simulink model "nms3D_2021"  (R2021a)
settings: Solver=ode15s  StartTime=0.0  StopTime=2  MaxStep=1e-2  RelTol=1e-2
StartFcn:
  | tic
StopFcn:
  | toc
  | 
  | 
  | %if GimbalLockFlag
  |  % fprintf(2, 'Almost reached Gimbal Lock of IMU. Simulation stopped.\n')
  | %end
  | 
  | %fprintf('Elapsed time: %4.2f sec (%4.2f%% realtime)\n', a, tout(end)/a*100)
values from neighbouring files (symbols this model uses):
  Balance02 = pMod(24:29)    [AssignSimulinkParams.m]    (also in assign_parameters.m = param(26:29))
  Balance13 = pMod(30:35)    [AssignSimulinkParams.m]    (also in assign_parameters.m = param(30:33))
  BalanceTrunk = pMod(22:23)    [AssignSimulinkParams.m]    (also in assign_parameters.m = param(22:23))
  BalanceTrunkLat = param(24:25)    [assign_parameters.m]
  BalanceTrunkLatOld = pMod(43:46)    [AssignSimulinkParams.m]    (also in assign_parameters.m = param(43:46))
  BalanceTrunkOld = param(49:53)    [assign_parameters.m]
  BasisStim = pMod(1:11)    [AssignSimulinkParams.m]    (also in assign_parameters.m = param(1:11))
  CompliantLeg = pMod(12:14)    [AssignSimulinkParams.m]    (also in assign_parameters.m = param(12:14))
  CompliantLegLat = pMod(15)    [AssignSimulinkParams.m]    (also in assign_parameters.m = param(15))
  PreventKneeOverextension = pMod(16:21)    [AssignSimulinkParams.m]    (also in assign_parameters.m = param(16:21))
  SwingCompLatOld = param(47:48)    [assign_parameters.m]
  Target02 = pMod(36:38)    [AssignSimulinkParams.m]    (also in assign_parameters.m = param(34:36))
  Target02_va = pMod(49:54)    [AssignSimulinkParams.m]    (also in assign_parameters.m = param(60:65))
  Target13 = pMod(39:41)    [AssignSimulinkParams.m]    (also in assign_parameters.m = param(37:39))
  Target13_va = pMod(55:60)    [AssignSimulinkParams.m]    (also in assign_parameters.m = param(66:71))
  theta0_world = param(59)    [assign_parameters.m]
  WramameiSL_1000 = readmatrix('WSL_1000_Norm_Sigmoid_MSE_cont.csv')    [nms3D_prep.m]
  ZramameiSL_1000 = readmatrix('ZSL_1000_Norm_Sigmoid_MSE_cont.csv')    [nms3D_prep.m]
undefined symbols (not defined in the file or in its folder): ICs, mParams, X, Y, Z
libraries: nesl_utility x106, sm_lib x87, simulink x70, eeGeneralControl x28, robotmaniplib x14, dspinverses x10, robotcorelib x5, dspmathops x3, vrlib x1, pid_lib x1
(part 1 of 8)
settings Model: Creator=hgeyer  LastModifiedBy=rachidramadan
settings SolverCC: AlgebraicLoopSolver=TrustRegion  MinimalZcImpactIntegration=on
settings OptimizationCC: EfficientMapNaN2IntZero=off
settings DebuggingCC: ReadBeforeWriteMsg=DisableAll  WriteAfterWriteMsg=DisableAll  WriteAfterReadMsg=DisableAll  IgnoredZcDiagnostic=none  MultiTaskDSMMsg=none  SFMachineParentedDataDiag=warning  ArithmeticOperatorsInVariantConditions=warning
settings HardwareCC: TargetBitPerLong=64  TargetBitPerPointer=64  TargetBitPerSizeT=64  TargetBitPerPtrDiffT=64  TargetLongLongMode=on  TargetIntDivRoundTo=Zero  TargetEndianess=LittleEndian  TargetWordSize=64  TargetHWDeviceType=MATLAB Host  ProdEqTarget=off
settings ModelReferenceCC: UpdateModelReferenceTargets=IfOutOfDate
settings SFSimCC: SFSimEcho=off  SimUseLocalCustomCode=off  CustomCodeUndefinedFunction=UseInterfaceOnly
settings CodeAppCC: MaxIdLength=128
settings ConfigComp: CovScope=ReferencedModels
settings SimscapeCC: SimscapeNormalizeSystem=off
settings ExplorerConfigSet: InternalSimMechanicsExplorerSettings="<ExplorerConfiguration><canonicalview>planar_xy</canonicalview><AnimationSetting><BasePlaybackSpeed>1.0</BasePlaybackSpeed><PlaybackSpeedFactor>1.0</PlaybackSpeedFactor></AnimationSetting><TilePanel><TileInfo><Tiles Columns=\"1\" Count=\"1\" Rows=\"1\"><Column Weight=\"1\"/><Row Weight=\"1\"/><Tile Height=\"1\" Width=\"1\" X=\"0\" Y=\"0\"/></Tiles></TileInfo><SceneInfo><SceneViewer><BGColor><R>0.60000002384185791</R><G>0.60000002384185791</G><B>0.60000002384185791</B></BGColor><Camera><DoPerspective>off</DoPerspective><Position><X>0.597774143722594631</X><Y>0.919449529340500282</Y><Z>14.1815791267909113</Z></Position><Center><X>0.597774143722594631</X><Y>0.919449529340500282</Y><Z>3.38181724401920292e-07</Z></Center><Up><X>0</X><Y>1</Y><Z>0</Z></Up><ViewLimDist>1</ViewLimDist><YLim>1.30566284997374105</YLim><XLim>1.60885047805753101</XLim></Camera></SceneViewer></SceneInfo></TilePanel><MechEditorPanel><Cameras/><GfxPanelCameraMap/><VideoCreator><PlaybackSpeedRatio>1.0</PlaybackSpeedRatio><FrameRate>30</FrameRate><VideoFormat>Motion JPEG AVI</VideoFormat><FrameSize>auto</FrameSize></VideoCreator></MechEditorPanel></ExplorerConfiguration>"

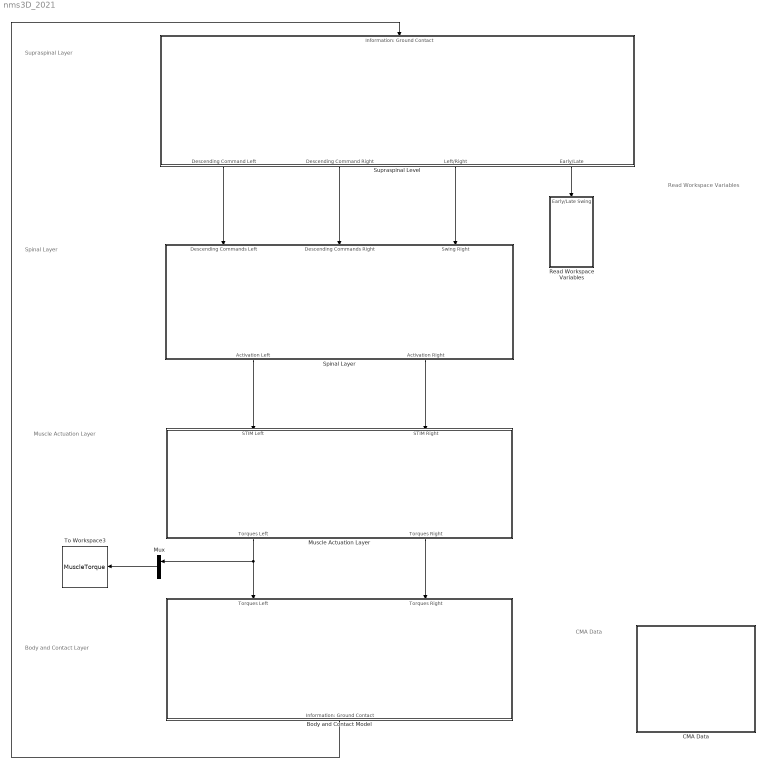
== system nms3D_2021 ==
  note: Spinal Layer
  note: Muscle Actuation Layer
  note: Body and Contact Layer
  note: Supraspinal Layer
  note: CMA Data
  note: Read Workspace Variables
  Body and Contact Model : Subsystem
  CMA Data : Subsystem
  Muscle Actuation Layer : Subsystem
  Mux : Mux  Inputs=2
  Read Workspace Variables : Subsystem
  Spinal Layer : Subsystem
  Supraspinal Level : Subsystem
  To Workspace3 : ToWorkspace  VariableName=MuscleTorque  SampleTime=-1
      settings: Save2DSignal=2-D array (concatenate along first dimension)
  wires:
  Spinal Layer/1(Activation Left) -> Muscle Actuation Layer/1(STIM Left)
  Spinal Layer/2(Activation Right) -> Muscle Actuation Layer/2(STIM Right)
  Supraspinal Level/1(Descending Command Left) -> Spinal Layer/1(Descending Commands Left)
  Supraspinal Level/2(Descending Command Right) -> Spinal Layer/2(Descending Commands Right)
  Body and Contact Model/1(Information: Ground Contact) -> Supraspinal Level/1(Information: Ground Contact)
  Mux/1 -> To Workspace3/1
  Muscle Actuation Layer/1(Torques Left) -> Body and Contact Model/1(Torques Left), Mux/1
  Supraspinal Level/3(Left/Right) -> Spinal Layer/3(Swing Right)
  Supraspinal Level/4(Early/Late) -> Read Workspace Variables/1(Early/Late Swing)
  Muscle Actuation Layer/2(Torques Right) -> Body and Contact Model/2(Torques Right)

== system nms3D_2021/Body and Contact Model ==
  note: Rigid Body
  note: Contact Model
  note: Vestibular System
  Torques Left : Inport
  Torques Right : Inport  Port=2
  6-DOF Joint IC : sm_lib/Joints/6-DOF Joint  JointMode=Normal  SenseConstraintForce=off  SenseConstraintForceX=off  SenseConstraintForceY=off  SenseConstraintForceZ=off  SenseConstraintTorque=off  SenseConstraintTorqueX=off  SenseConstraintTorqueY=off  SenseConstraintTorqueZ=off  SenseTotalForce=off  SenseTotalForceX=off  SenseTotalForceY=off  SenseTotalForceZ=off  SenseTotalTorque=off  SenseTotalTorqueX=off  SenseTotalTorqueY=off  SenseTotalTorqueZ=off  CompositeWrenchDir=BaseOnFollower  CompositeWrenchFrame=FollowerFrame  PxEquilibriumPosition=0  PxEquilibriumPositionUnits=m  PxSpringStiffness=0  PxSpringStiffnessUnits=N/m  PxDampingCoefficient=0  PxDampingCoefficientUnits=N/(m/s)  PxTorqueActuationMode=NoTorque  PxMotionActuationMode=ComputedMotion  PxSensePosition=off  PxSenseVelocity=off  PxSenseAcceleration=off  PxSenseTorqueForce=off  PxSenseLowerLimitTorqueForce=off  PxSenseUpperLimitTorqueForce=off  PxLowerLimitSpecify=off  PxLowerLimitBound=-1  PxLowerLimitBoundUnits=m  PxLowerLimitStiffness=1e6  PxLowerLimitStiffnessUnits=N/m  PxLowerLimitDamping=1e3  PxLowerLimitDampingUnits=N/(m/s)  PxLowerLimitTransitionRegionWidth=1e-4  PxLowerLimitTransitionRegionWidthUnits=m  PxUpperLimitSpecify=off  PxUpperLimitBound=1  PxUpperLimitBoundUnits=m  PxUpperLimitStiffness=1e6  PxUpperLimitStiffnessUnits=N/m  PxUpperLimitDamping=1e3  PxUpperLimitDampingUnits=N/(m/s)  PxUpperLimitTransitionRegionWidth=1e-4  PxUpperLimitTransitionRegionWidthUnits=m  PxPositionTargetSpecify=on  PxPositionTargetPriority=High  PxPositionTargetValue=ICs.trunk.x0  PxPositionTargetValueUnits=m  PxVelocityTargetSpecify=on  PxVelocityTargetPriority=High  PxVelocityTargetValue=ICs.trunk.vx0  PxVelocityTargetValueUnits=m/s  PyEquilibriumPosition=0  PyEquilibriumPositionUnits=m  PySpringStiffness=0  PySpringStiffnessUnits=N/m  PyDampingCoefficient=0  PyDampingCoefficientUnits=N/(m/s)  PyTorqueActuationMode=NoTorque  PyMotionActuationMode=ComputedMotion  PySensePosition=off  PySenseVelocity=off  PySenseAcceleration=off  PySenseTorqueForce=off  PySenseLowerLimitTorqueForce=off  PySenseUpperLimitTorqueForce=off  PyLowerLimitSpecify=off  PyLowerLimitBound=-1  PyLowerLimitBoundUnits=m  PyLowerLimitStiffness=1e6  PyLowerLimitStiffnessUnits=N/m  PyLowerLimitDamping=1e3  PyLowerLimitDampingUnits=N/(m/s)  PyLowerLimitTransitionRegionWidth=1e-4  PyLowerLimitTransitionRegionWidthUnits=m  PyUpperLimitSpecify=off  PyUpperLimitBound=1  PyUpperLimitBoundUnits=m  PyUpperLimitStiffness=1e6  PyUpperLimitStiffnessUnits=N/m  PyUpperLimitDamping=1e3  PyUpperLimitDampingUnits=N/(m/s)  PyUpperLimitTransitionRegionWidth=1e-4  PyUpperLimitTransitionRegionWidthUnits=m  PyPositionTargetSpecify=on  PyPositionTargetPriority=High  PyPositionTargetValue=ICs.trunk.y0  PyPositionTargetValueUnits=m  PyVelocityTargetSpecify=off  PyVelocityTargetPriority=High  PyVelocityTargetValue=0  PyVelocityTargetValueUnits=m/s  PzEquilibriumPosition=0  PzEquilibriumPositionUnits=m  PzSpringStiffness=0  PzSpringStiffnessUnits=N/m  PzDampingCoefficient=0  PzDampingCoefficientUnits=N/(m/s)  PzTorqueActuationMode=NoTorque  PzMotionActuationMode=ComputedMotion  PzSensePosition=off  PzSenseVelocity=off  PzSenseAcceleration=off  PzSenseTorqueForce=off  PzSenseLowerLimitTorqueForce=off  PzSenseUpperLimitTorqueForce=off  PzLowerLimitSpecify=off  PzLowerLimitBound=-1  PzLowerLimitBoundUnits=m  PzLowerLimitStiffness=1e6  PzLowerLimitStiffnessUnits=N/m  PzLowerLimitDamping=1e3  PzLowerLimitDampingUnits=N/(m/s)  PzLowerLimitTransitionRegionWidth=1e-4  PzLowerLimitTransitionRegionWidthUnits=m  PzUpperLimitSpecify=off  PzUpperLimitBound=1  PzUpperLimitBoundUnits=m  PzUpperLimitStiffness=1e6  PzUpperLimitStiffnessUnits=N/m  PzUpperLimitDamping=1e3  PzUpperLimitDampingUnits=N/(m/s)  PzUpperLimitTransitionRegionWidth=1e-4  PzUpperLimitTransitionRegionWidthUnits=m  PzPositionTargetSpecify=on  PzPositionTargetPriority=High  PzPositionTargetValue=ICs.trunk.z0  PzPositionTargetValueUnits=m  PzVelocityTargetSpecify=on  PzVelocityTargetPriority=High  PzVelocityTargetValue=ICs.trunk.vz0  PzVelocityTargetValueUnits=m/s  SphDefPosRotationMethod=None  SphDefPosRotationAngleUnits=deg  SphDefPosRotationStandardAxis=+Z  SphDefPosRotationAngle=0.0  SphDefPosRotationArbitraryAxis=[0 0 1]  SphDefPosFollAlignAxisA=+X  SphDefPosBaseAlignAxisA=+Y  SphDefPosFollAlignAxisB=+Y  SphDefPosBaseAlignAxisB=+Z  SphDefPosRotationSequenceAxes=FollowerAxes  SphDefPosRotationSequence=XYX  SphDefPosRotationSequenceAngles=[0 0 0]  SphDefPosRotationSequenceAnglesUnits=deg  SphDefPosRotationMatrix=[1 0 0; 0 1 0; 0 0 1]  SphEqPosRotationMethod=None  SphEqPosRotationAngleUnits=deg  SphEqPosRotationStandardAxis=+Y  SphEqPosRotationAngle=0.0  SphEqPosRotationArbitraryAxis=[0 0 1]  SphEqPosFollAlignAxisA=+X  SphEqPosBaseAlignAxisA=+Y  SphEqPosFollAlignAxisB=+Y  SphEqPosBaseAlignAxisB=+Z  SphEqPosRotationSequenceAxes=FollowerAxes  SphEqPosRotationSequence=XYZ  SphEqPosRotationSequenceAngles=[0 0 -0.3]  SphEqPosRotationSequenceAnglesUnits=rad  SphEqPosRotationMatrix=[1 0 0; 0 1 0; 0 0 1]  SphSpringStiffness=0  SphSpringStiffnessUnits=N*m/deg  SphDampingCoefficient=0  SphDampingCoefficientUnits=N*m/(deg/s)  SphActuateTorqueX=off  SphActuateTorqueY=off  SphActuateTorqueZ=off  SphActuateTorque=on  SphTorqueActuationMode=NoTorque  SphMotionActuationMode=ComputedMotion  SphActuationFrame=BaseFrame  SphSensePosition=off  SphSenseVelocityX=off  SphSenseVelocityY=off  SphSenseVelocityZ=off  SphSenseVelocity=off  SphSenseAccelerationX=off  SphSenseAccelerationY=off  SphSenseAccelerationZ=off  SphSenseAcceleration=off  SphSenseTorqueX=off  SphSenseTorqueY=off  SphSenseTorqueZ=off  SphSenseTorqueForce=off  SphSenseLowerLimitTorqueMag=off  SphSenseUpperLimitTorqueMag=off  SphSensingFrame=BaseFrame  SphLowerLimitSpecify=off  SphLowerLimitBound=15  SphLowerLimitBoundUnits=deg  SphLowerLimitStiffness=1e4  SphLowerLimitStiffnessUnits=N*m/deg  SphLowerLimitDamping=10  SphLowerLimitDampingUnits=N*m/(deg/s)  SphLowerLimitTransitionRegionWidth=0.1  SphLowerLimitTransitionRegionWidthUnits=deg  SphUpperLimitSpecify=off  SphUpperLimitBound=45  SphUpperLimitBoundUnits=deg  SphUpperLimitStiffness=1e4  SphUpperLimitStiffnessUnits=N*m/deg  SphUpperLimitDamping=10  SphUpperLimitDampingUnits=N*m/(deg/s)  SphUpperLimitTransitionRegionWidth=0.1  SphUpperLimitTransitionRegionWidthUnits=deg  SphPositionTargetRotationMethod=RotationSequence  SphPositionTargetRotationAngleUnits=deg  SphPositionTargetRotationStandardAxis=+Z  SphPositionTargetRotationAngle=0.0  SphPositionTargetRotationArbitraryAxis=[0 0 1]  SphPositionTargetFollAlignAxisA=+X  SphPositionTargetBaseAlignAxisA=+Y  SphPositionTargetFollAlignAxisB=+Y  SphPositionTargetBaseAlignAxisB=+Z  SphPositionTargetRotationSequenceAxes=BaseAxes  SphPositionTargetRotationSequence=XZY  SphPositionTargetRotationSequenceAngles=[ICs.trunk.qR0 ICs.trunk.qP0 ICs.trunk.qY0 ]  SphPositionTargetRotationSequenceAnglesUnits=rad  SphPositionTargetRotationMatrix=[1 0 0; 0 1 0; 0 0 1]  SphPositionTargetSpecify=on  SphPositionTargetPriority=High  SphVelocityTargetValue=[ICs.trunk.qR0 ICs.trunk.qP0 ICs.trunk.qY0 ]  SphVelocityTargetValueUnits=deg/s  SphVelocityTargetSpecify=on  SphVelocityTargetPriority=High  SphVelocityTargetInFollowerFrame=on
  L Leg : Subsystem
  R Leg : Subsystem
  Subsystem : Subsystem
  Terminator : Terminator
  Terminator1 : Terminator
  Trunk (floating base) : Subsystem
  Vestibular System : Subsystem
  World Frame : Subsystem
  Information: Ground Contact : Outport
  tag scope: Llegddq=global, Llegdq=global, Llegq=global, Rlegddq=global, Rlegdq=global, Rlegq=global
  wires:
  R Leg/2(Position Right Ankle [m]) -> Vestibular System/1(Ankle Position Right [m])
  L Leg/2(" Position Left Ankle [m]") -> Vestibular System/2(Ankle Position Left [m])
  Subsystem/1(Information: Ground Contact) -> Information: Ground Contact/1
  L Leg/1(Rotation Matrix Left Knee (world)) -> Terminator/1
  R Leg/1(Rotation Matrix Right Knee (World)) -> Terminator1/1
  Torques Right/1 -> R Leg/1(Torques [Nm])
  Torques Left/1 -> L Leg/1(Torques [Nm])
  L Leg/3(Joint Angles Left [rad]) -> [Llegq]
  L Leg/4("Joint Velocities Left [rad/s] ") -> [Llegdq]
  L Leg/5(Joint Accelerations Left [rad/s^2]) -> [Llegddq]
  R Leg/3(Joint Angles Right [rad]) -> [Rlegq]
  R Leg/4("Joint Velocities Right [rad/s] ") -> [Rlegdq]
  R Leg/5(Joint Accelerations Right [rad/s^2]) -> [Rlegddq]
  connections:
  Trunk (floating base)/RConn1 -- Vestibular System/LConn3 -- L Leg/LConn1
  World Frame/RConn1 -- Subsystem/LConn1 -- 6-DOF Joint IC/LConn1
  L Leg/RConn1 -- Subsystem/RConn1
  L Leg/RConn2 -- Subsystem/RConn2
  L Leg/RConn3 -- Subsystem/RConn3
  L Leg/RConn4 -- Subsystem/RConn4
  R Leg/RConn3 -- Subsystem/RConn7
  R Leg/RConn4 -- Subsystem/RConn8
  Vestibular System/LConn2 -- R Leg/LConn1 -- Trunk (floating base)/RConn2
  6-DOF Joint IC/RConn1 -- Vestibular System/LConn1 -- Trunk (floating base)/LConn1
  Subsystem/RConn6 -- R Leg/RConn1
  R Leg/RConn2 -- Subsystem/RConn5

== system nms3D_2021/CMA Data ==
  note: The output of SS_dist yields the relative distance of the limb.
  Mux : Mux  Inputs=7
  SS_dist1 : Subsystem  TreatAsAtomicUnit=on
  Step Counter : Subsystem
  check steady state : Subsystem
  wires:
  Step Counter/1(nStep) -> check steady state/2(nStep)
  [Contact_left] -> Step Counter/2(Step1), SS_dist1/Trigger
  [Contact_right] -> Step Counter/1(Step2)
  [Ball_right] -> Mux/1
  [AnklePosR] -> Mux/2
  [HipR] -> Mux/3
  [TRK_CG] -> Mux/4
  [HipL] -> Mux/5
  [Ball_left] -> Mux/6
  [AnklePosL] -> Mux/7
  Mux/1 -> check steady state/1(p)
  check steady state/1(SS_dist) -> SS_dist1/1(In1)

== system nms3D_2021/Muscle Actuation Layer ==
  note: Muscle Actuation Layer
  STIM Left : Inport
  STIM Right : Inport  Port=2
  Muscles Left : Subsystem
  Muscles Right : Subsystem
  Mux : Mux  Inputs=5
  Mux1 : Mux  Inputs=5
  Terminator : Terminator
  Terminator1 : Terminator
  Torques Left : Outport
  Torques Right : Outport  Port=2
  wires:
  STIM Left/1 -> Muscles Left/1(STIM Left)
  STIM Right/1 -> Muscles Right/1(STIM Right)
  Muscles Left/1(tauHipPitchL) -> Mux/1
  Muscles Left/2(tauHipRollL) -> Mux/2
  Muscles Left/3(tauKneeL) -> Mux/3
  Mux/1 -> Torques Left/1
  Mux1/1 -> Torques Right/1
  Muscles Left/5(tauAnklePitchL) -> Mux/5
  Muscles Left/4(tauAnkleRollL) -> Mux/4
  Muscles Right/1(tauHipPitchR) -> Mux1/1
  Muscles Right/2(tauHipRollR) -> Mux1/2
  Muscles Right/3(tauKneeR) -> Mux1/3
  Muscles Right/4(tauHipAnkleRollR) -> Mux1/4
  Muscles Right/5(tauHipAnklePitchR) -> Mux1/5
  Muscles Left/6("Leg Torque ") -> Terminator/1
  Muscles Right/6(Leg Torque) -> Terminator1/1

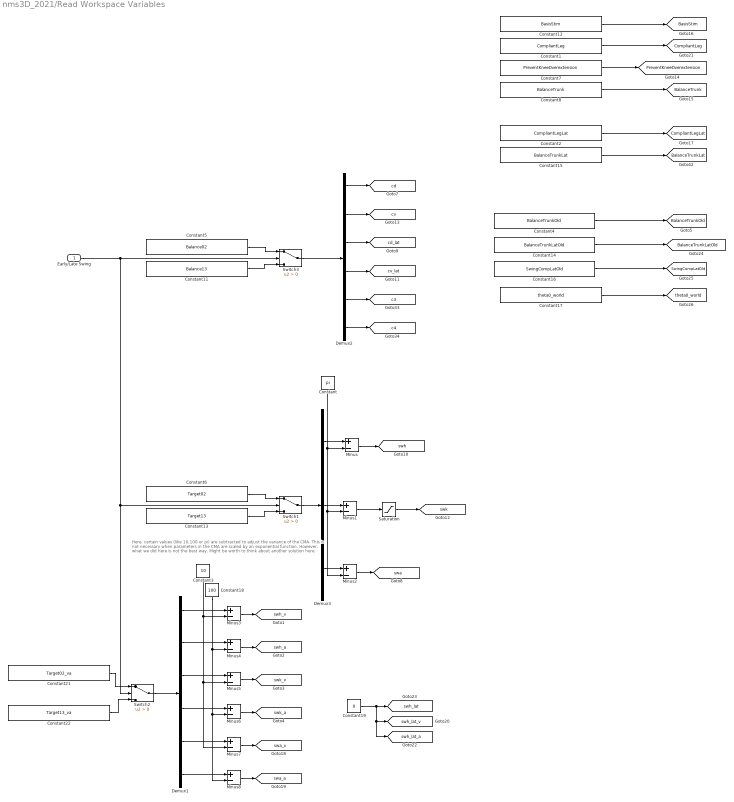
== system nms3D_2021/Read Workspace Variables ==
  note: Here, certain values (like 10,100 or pi) are subtracted to adjust the variance of the CMA.
      | This is not necessary when  parameters in the CMA are scaled by an exponential function. However, what we did here is not the best way. Might be worth to think about another solution here.
  Early/Late Swing : Inport
  Constant : Constant  Value=pi
  Constant1 : Constant  Value=CompliantLeg
  Constant11 : Constant  Value=Balance13
  Constant12 : Constant  Value=BasisStim
  Constant13 : Constant  Value=Target13
  Constant14 : Constant  Value=BalanceTrunkLatOld
  Constant15 : Constant  Value=BalanceTrunkLat
  Constant16 : Constant  Value=SwingCompLatOld
  Constant17 : Constant  Value=theta0_world
  Constant18 : Constant  Value=100
  Constant19 : Constant  Value=0
  Constant2 : Constant  Value=CompliantLegLat
  Constant21 : Constant  Value=Target02_va
  Constant22 : Constant  Value=Target13_va
  Constant3 : Constant  Value=10
  Constant4 : Constant  Value=BalanceTrunkOld
  Constant5 : Constant  Value=Balance02
  Constant6 : Constant  Value=Target02
  Constant7 : Constant  Value=PreventKneeOverextension
  Constant8 : Constant  Value=BalanceTrunk
  Demux1 : Demux  Outputs=6
  Demux2 : Demux  Outputs=6
  Demux3 : Demux  Outputs=3
  Minus{,1..8} (9 alike) : Sum  Inputs=+-
  Saturation : Saturate  UpperLimit=pi  LowerLimit=0
  Switch1 : Switch  Criteria=u2 > Threshold  ZeroCross=off
  Switch2 : Switch  Criteria=u2 > Threshold
  Switch3 : Switch  Criteria=u2 > Threshold  ZeroCross=off
  tag scope: BalanceTrunk=global, BalanceTrunkLat=global, BalanceTrunkLatOld=global, BalanceTrunkOld=global, BasisStim=global, CompliantLeg=global, CompliantLegLat=global, PreventKneeOverextension=global, SwingCompLatOld=global, c3=global, c4=global, cd=global, cd_lat=global, cv=global, cv_lat=global, swa=global, swa_a=global, swa_v=global, swh=global, swh_a=global, swh_lat=global, swh_lat_a=global, swh_lat_v=global, swh_v=global, swk=global, swk_a=global, swk_v=global, theta0_world=global
  wires:
  Constant1/1 -> [CompliantLeg]
  Constant8/1 -> [BalanceTrunk]
  Constant15/1 -> [BalanceTrunkLat]
  Constant12/1 -> [BasisStim]
  Constant7/1 -> [PreventKneeOverextension]
  Switch1/1 -> Demux3/1
  Constant5/1 -> Switch3/1
  Demux2/3 -> [cd_lat]
  Demux2/2 -> [cv]
  Switch3/1 -> Demux2/1
  Demux2/4 -> [cv_lat]
  Demux2/1 -> [cd]
  Constant11/1 -> Switch3/3
  Constant6/1 -> Switch1/1
  Constant13/1 -> Switch1/3
  Constant2/1 -> [CompliantLegLat]
  Minus/1 -> [swh]
  Demux3/1 -> Minus/1
  Minus1/1 -> Saturation/1
  Demux3/2 -> Minus1/1
  Minus2/1 -> [swa]
  Demux3/3 -> Minus2/1
  Constant/1 -> Minus/2, Minus1/2, Minus2/2
  Constant4/1 -> [BalanceTrunkOld]
  Constant14/1 -> [BalanceTrunkLatOld]
  Constant16/1 -> [SwingCompLatOld]
  Constant17/1 -> [theta0_world]
  Early/Late Swing/1 -> Switch2/2, Switch1/2, Switch3/2
  Constant19/1 -> [swh_lat], [swh_lat_v], [swh_lat_a]
  Switch2/1 -> Demux1/1
  Constant21/1 -> Switch2/1
  Constant22/1 -> Switch2/3
  Minus3/1 -> [swh_v]
  Minus4/1 -> [swh_a]
  Minus5/1 -> [swk_v]
  Minus6/1 -> [swk_a]
  Minus7/1 -> [swa_v]
  Minus8/1 -> [swa_a]
  Demux1/6 -> Minus8/1
  Demux1/5 -> Minus7/1
  Demux1/4 -> Minus6/1
  Demux1/3 -> Minus5/1
  Demux1/2 -> Minus4/1
  Demux1/1 -> Minus3/1
  Constant3/1 -> Minus3/2, Minus5/2, Minus7/2
  Constant18/1 -> Minus4/2, Minus6/2, Minus8/2
  Demux2/5 -> [c3]
  Demux2/6 -> [c4]
  Saturation/1 -> [swk]

== system nms3D_2021/Spinal Layer ==
  Descending Commands Left : Inport
  Descending Commands Right : Inport  Port=2
  Swing Right : Inport  Port=3
  Add1 : Sum
  Add2 : Sum
  Gain : Gain
  Gain1 : Gain
  Saturation1 : Saturate  UpperLimit=1  LowerLimit=0.001  ZeroCross=off
  Saturation2 : Saturate  UpperLimit=1  LowerLimit=0.001  ZeroCross=off
  Spinal Reflexes Control Left (Stance only) : Subsystem
  Spinal Reflexes Control Right (Stance only) : Subsystem
  Stretch Reflex : Subsystem
  Switch : Switch  Criteria=u2 > Threshold
  Switch1 : Switch  Criteria=u2 > Threshold
  Activation Left : Outport
  Activation Right : Outport  Port=2
  wires:
  Descending Commands Right/1 -> Stretch Reflex/2(Descending Commands Right)
  Descending Commands Left/1 -> Stretch Reflex/1(Descending Commands Left)
  Swing Right/1 -> Switch/2, Spinal Reflexes Control Right (Stance only)/1(Left/Right), Spinal Reflexes Control Left (Stance only)/1(Left/Right), Switch1/2
  Spinal Reflexes Control Left (Stance only)/1(Activation Left) -> Add1/2
  Spinal Reflexes Control Right (Stance only)/1(Activation Right) -> Add2/2
  Switch1/1 -> Saturation1/1
  Switch/1 -> Saturation2/1
  Add1/1 -> Switch1/1
  Add2/1 -> Switch/3
  Stretch Reflex/2(Activation Right) -> Gain/1, Switch/1
  Stretch Reflex/1(Activation Left) -> Spinal Reflexes Control Right (Stance only)/2(Activation Swing Left), Gain1/1, Switch1/3
  Saturation1/1 -> Activation Left/1
  Saturation2/1 -> Activation Right/1
  Gain/1 -> Add2/1
  Gain1/1 -> Add1/1

== system nms3D_2021/Supraspinal Level ==
  note: Finite State Machine
  note: Computing Descending Commands for Swing Leg Control
  Information: Ground Contact : Inport
  Early/ Late : Logic  Operator=OR  AllPortsSameDT=off  OutDataTypeStr=boolean
  Finite State Machine : Subsystem
  Left/ Right : Logic  Operator=OR  AllPortsSameDT=off  OutDataTypeStr=boolean
  Subsystem : Subsystem
  Terminator : Terminator
  To Workspace1 : ToWorkspace  VariableName=LateRight  SampleTime=-1
      settings: Save2DSignal=2-D array (concatenate along first dimension)
  To Workspace2 : ToWorkspace  VariableName=EarlyRight  SampleTime=-1
      settings: Save2DSignal=2-D array (concatenate along first dimension)
  To Workspace3 : ToWorkspace  VariableName=EarlyLeft  SampleTime=-1
      settings: Save2DSignal=2-D array (concatenate along first dimension)
  To Workspace4 : ToWorkspace  VariableName=Contact  SampleTime=-1
      settings: Save2DSignal=2-D array (concatenate along first dimension)
  Descending Command Left : Outport
  Descending Command Right : Outport  Port=2
  Left/Right : Outport  Port=3
  Early/Late : Outport  Port=4
  wires:
  Finite State Machine/3(Early Left Swing) -> To Workspace3/1, Early/ Late/2
  Finite State Machine/1(Early Right Swing) -> To Workspace2/1, Left/ Right/1, Early/ Late/1
  Finite State Machine/4(Late Left Swing) -> Terminator/1
  Finite State Machine/2(Late Right Swing) -> To Workspace1/1, Left/ Right/2
  Early/ Late/1 -> Subsystem/1(Early/Late Swing), Early/Late/1
  Information: Ground Contact/1 -> To Workspace4/1, Finite State Machine/1(Information: Ground Contact)
  Subsystem/1(Descending Command Left) -> Descending Command Left/1
  Subsystem/2(Descending Command Right) -> Descending Command Right/1
  Left/ Right/1 -> Subsystem/2(Swing Right), Left/Right/1

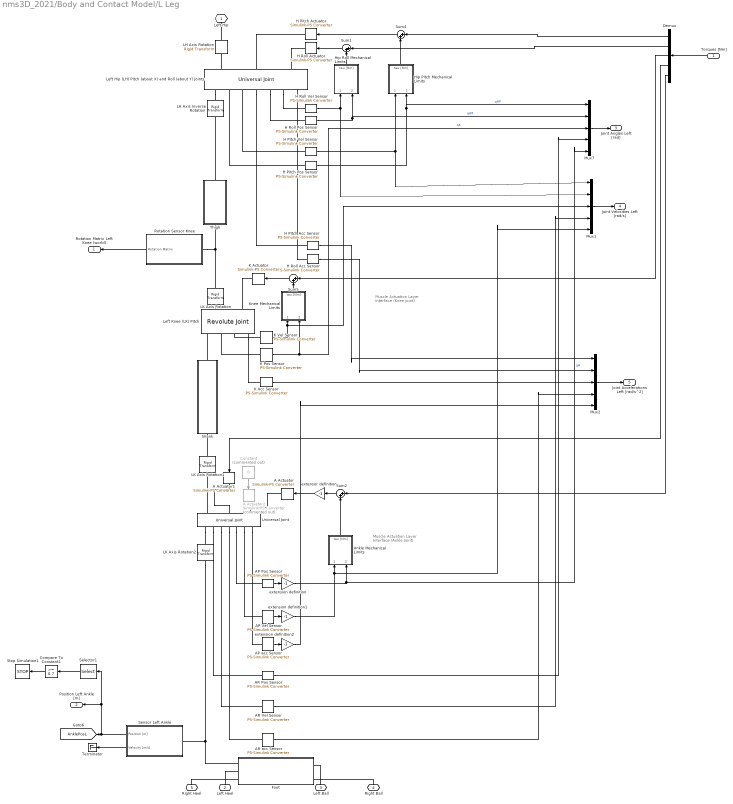
== system nms3D_2021/Body and Contact Model/L Leg ==
  note: Muscle Actuation
      | Layer Interface
      | (Ankle Joint)
  note: Muscle Actuation
      | Layer Interface
      | (Knee Joint)
  Torques [Nm] : Inport
  " K Actuator" : nesl_utility/Simulink-PS Converter  PhysicalDomain=network_engine_domain  SubClassName=ps_input  LeftPortType=input  RightPortType=output  PseudoPeriodic=off  Frequencies=[]  NoiseDistribution=none  NoiseParameters=[]  Unit=N*m  AffineConversion=off  FilteringAndDerivatives=zero  SimscapeFilterOrder=1  InputFilterTimeConstant=.001  UdotUserProvided=0
      settings: SourceProductBaseCode=PW,SS
  A Actuator : nesl_utility/Simulink-PS Converter  PhysicalDomain=network_engine_domain  SubClassName=ps_input  LeftPortType=input  RightPortType=output  PseudoPeriodic=off  Frequencies=[]  NoiseDistribution=none  NoiseParameters=[]  Unit=N*m  AffineConversion=off  FilteringAndDerivatives=zero  SimscapeFilterOrder=1  InputFilterTimeConstant=.001  UdotUserProvided=0
      settings: SourceProductBaseCode=PW,SS
  A Actuator1 : nesl_utility/Simulink-PS Converter  PhysicalDomain=network_engine_domain  SubClassName=ps_input  LeftPortType=input  RightPortType=output  PseudoPeriodic=off  Frequencies=[]  NoiseDistribution=none  NoiseParameters=[]  Unit=N*m  AffineConversion=off  FilteringAndDerivatives=zero  SimscapeFilterOrder=1  InputFilterTimeConstant=.001  UdotUserProvided=0
      settings: SourceProductBaseCode=PW,SS
  A Actuator2 : nesl_utility/Simulink-PS Converter  Commented=on  PhysicalDomain=network_engine_domain  SubClassName=ps_input  LeftPortType=input  RightPortType=output  PseudoPeriodic=off  Frequencies=[]  NoiseDistribution=none  NoiseParameters=[]  Unit=rad  AffineConversion=off  FilteringAndDerivatives=zero  SimscapeFilterOrder=1  InputFilterTimeConstant=.001  UdotUserProvided=0
      settings: SourceProductBaseCode=PW,SS
  AP Pos Sensor : nesl_utility/PS-Simulink Converter  PhysicalDomain=network_engine_domain  SubClassName=ps_output  LeftPortType=input  RightPortType=output  PseudoPeriodic=off  Frequencies=[]  Unit=rad  AffineConversion=off
      settings: SourceProductBaseCode=PW,SS
  AP Vel Sensor : nesl_utility/PS-Simulink Converter  PhysicalDomain=network_engine_domain  SubClassName=ps_output  LeftPortType=input  RightPortType=output  PseudoPeriodic=off  Frequencies=[]  Unit=rad/s  AffineConversion=off
      settings: SourceProductBaseCode=PW,SS
  AP acc Sensor : nesl_utility/PS-Simulink Converter  PhysicalDomain=network_engine_domain  SubClassName=ps_output  LeftPortType=input  RightPortType=output  PseudoPeriodic=off  Frequencies=[]  Unit=rad/(s^2)  AffineConversion=off
      settings: SourceProductBaseCode=PW,SS
  AR Pos Sensor : nesl_utility/PS-Simulink Converter  PhysicalDomain=network_engine_domain  SubClassName=ps_output  LeftPortType=input  RightPortType=output  PseudoPeriodic=off  Frequencies=[]  Unit=rad  AffineConversion=off
      settings: SourceProductBaseCode=PW,SS
  AR Vel Sensor : nesl_utility/PS-Simulink Converter  PhysicalDomain=network_engine_domain  SubClassName=ps_output  LeftPortType=input  RightPortType=output  PseudoPeriodic=off  Frequencies=[]  Unit=rad/s  AffineConversion=off
      settings: SourceProductBaseCode=PW,SS
  AR acc Sensor : nesl_utility/PS-Simulink Converter  PhysicalDomain=network_engine_domain  SubClassName=ps_output  LeftPortType=input  RightPortType=output  PseudoPeriodic=off  Frequencies=[]  Unit=rad/(s^2)  AffineConversion=off
      settings: SourceProductBaseCode=PW,SS
  Ankle Mechanical Limits : Subsystem
  Compare To Constant1 : simulink/Logic and Bit Operations/Compare To Constant  relop=>=  const=0.7  OutDataTypeStr=boolean
  Constant : Constant  Commented=on  Value=0
  Demux : Demux  Outputs=5
  Foot : Subsystem
  H Pitch Actuator : nesl_utility/Simulink-PS Converter  PhysicalDomain=network_engine_domain  SubClassName=ps_input  LeftPortType=input  RightPortType=output  PseudoPeriodic=off  Frequencies=[]  NoiseDistribution=none  NoiseParameters=[]  Unit=N*m  AffineConversion=off  FilteringAndDerivatives=zero  SimscapeFilterOrder=1  InputFilterTimeConstant=.001  UdotUserProvided=0
      settings: SourceProductBaseCode=PW,SS
  H Pitch Acc Sensor : nesl_utility/PS-Simulink Converter  PhysicalDomain=network_engine_domain  SubClassName=ps_output  LeftPortType=input  RightPortType=output  PseudoPeriodic=off  Frequencies=[]  Unit=rad/(s^2)  AffineConversion=off
      settings: SourceProductBaseCode=PW,SS
  H Pitch Pos Sensor : nesl_utility/PS-Simulink Converter  PhysicalDomain=network_engine_domain  SubClassName=ps_output  LeftPortType=input  RightPortType=output  PseudoPeriodic=off  Frequencies=[]  Unit=rad  AffineConversion=off
      settings: SourceProductBaseCode=PW,SS
  H Pitch Vel Sensor : nesl_utility/PS-Simulink Converter  PhysicalDomain=network_engine_domain  SubClassName=ps_output  LeftPortType=input  RightPortType=output  PseudoPeriodic=off  Frequencies=[]  Unit=rad/s  AffineConversion=off
      settings: SourceProductBaseCode=PW,SS
  H Roll Actuator : nesl_utility/Simulink-PS Converter  PhysicalDomain=network_engine_domain  SubClassName=ps_input  LeftPortType=input  RightPortType=output  PseudoPeriodic=off  Frequencies=[]  NoiseDistribution=none  NoiseParameters=[]  Unit=N*m  AffineConversion=off  FilteringAndDerivatives=zero  SimscapeFilterOrder=1  InputFilterTimeConstant=.001  UdotUserProvided=0
      settings: SourceProductBaseCode=PW,SS
  H Roll Acc Sensor : nesl_utility/PS-Simulink Converter  PhysicalDomain=network_engine_domain  SubClassName=ps_output  LeftPortType=input  RightPortType=output  PseudoPeriodic=off  Frequencies=[]  Unit=rad/(s^2)  AffineConversion=off
      settings: SourceProductBaseCode=PW,SS
  H Roll Pos Sensor : nesl_utility/PS-Simulink Converter  PhysicalDomain=network_engine_domain  SubClassName=ps_output  LeftPortType=input  RightPortType=output  PseudoPeriodic=off  Frequencies=[]  Unit=rad  AffineConversion=off
      settings: SourceProductBaseCode=PW,SS
  "H Roll Vel Sensor " : nesl_utility/PS-Simulink Converter  PhysicalDomain=network_engine_domain  SubClassName=ps_output  LeftPortType=input  RightPortType=output  PseudoPeriodic=off  Frequencies=[]  Unit=rad/s  AffineConversion=off
      settings: SourceProductBaseCode=PW,SS
  Hip Pitch Mechanical Limits : Subsystem
  Hip Roll Mechanical Limits : Subsystem
  K Acc Sensor : nesl_utility/PS-Simulink Converter  PhysicalDomain=network_engine_domain  SubClassName=ps_output  LeftPortType=input  RightPortType=output  PseudoPeriodic=off  Frequencies=[]  Unit=rad/(s^2)  AffineConversion=off
      settings: SourceProductBaseCode=PW,SS
  K Pos Sensor : nesl_utility/PS-Simulink Converter  PhysicalDomain=network_engine_domain  SubClassName=ps_output  LeftPortType=input  RightPortType=output  PseudoPeriodic=off  Frequencies=[]  Unit=rad  AffineConversion=off
      settings: SourceProductBaseCode=PW,SS
  K Vel Sensor : nesl_utility/PS-Simulink Converter  PhysicalDomain=network_engine_domain  SubClassName=ps_output  LeftPortType=input  RightPortType=output  PseudoPeriodic=off  Frequencies=[]  Unit=rad/s  AffineConversion=off
      settings: SourceProductBaseCode=PW,SS
  Knee Mechanical Limits : Subsystem
  LH Axis Inverse Rotation : sm_lib/Frames and Transforms/Rigid Transform  TranslationMethod=None  TranslationStandardOffset=-0.2  TranslationLengthUnit=m  TranslationStandardAxis=+Y  TranslationCartesianOffset=0  TranslationROffset=0  TranslationROffsetUnits=m  TranslationZOffset=0  TranslationZOffsetUnits=m  TranslationThetaOffset=0  TranslationThetaOffsetUnits=deg  RotationMethod=RotationSequence  RotationAngleUnits=deg  RotationStandardAxis=+X  RotationAngle=-90  RotationArbitraryAxis=[0 0 1]  FollAlignAxisA=+X  BaseAlignAxisA=+Y  FollAlignAxisB=+Y  BaseAlignAxisB=+Z  RotationSequenceAxes=BaseAxes  RotationSequence=YXY  RotationSequenceAngles=[-90 -90 0]  RotationSequenceAnglesUnits=deg  RotationMatrix=[1 0 0; 0 1 0; 0 0 1]
  LH Axis Rotation : sm_lib/Frames and Transforms/Rigid Transform  TranslationMethod=None  TranslationStandardOffset=-0.2  TranslationLengthUnit=m  TranslationStandardAxis=+Y  TranslationCartesianOffset=0  TranslationROffset=0  TranslationROffsetUnits=m  TranslationZOffset=0  TranslationZOffsetUnits=m  TranslationThetaOffset=0  TranslationThetaOffsetUnits=deg  RotationMethod=RotationSequence  RotationAngleUnits=deg  RotationStandardAxis=+X  RotationAngle=90  RotationArbitraryAxis=[0 0 1]  FollAlignAxisA=+X  BaseAlignAxisA=+Y  FollAlignAxisB=+Y  BaseAlignAxisB=+Z  RotationSequenceAxes=FollowerAxes  RotationSequence=XZX  RotationSequenceAngles=[-90 90 0]  RotationSequenceAnglesUnits=deg  RotationMatrix=[1 0 0; 0 1 0; 0 0 1]
  LK Axis Rotation : sm_lib/Frames and Transforms/Rigid Transform  TranslationMethod=None  TranslationStandardOffset=-0.5  TranslationLengthUnit=m  TranslationStandardAxis=+Y  TranslationCartesianOffset=0  TranslationROffset=0  TranslationROffsetUnits=m  TranslationZOffset=0  TranslationZOffsetUnits=m  TranslationThetaOffset=0  TranslationThetaOffsetUnits=deg  RotationMethod=RotationSequence  RotationAngleUnits=deg  RotationStandardAxis=+X  RotationAngle=-90  RotationArbitraryAxis=[0 0 1]  FollAlignAxisA=+X  BaseAlignAxisA=+Y  FollAlignAxisB=+Y  BaseAlignAxisB=+Z  RotationSequenceAxes=BaseAxes  RotationSequence=ZXZ  RotationSequenceAngles=[180 0 0]  RotationSequenceAnglesUnits=deg  RotationMatrix=[1 0 0; 0 1 0; 0 0 1]
  LK Axis Rotation1 : sm_lib/Frames and Transforms/Rigid Transform  TranslationMethod=None  TranslationStandardOffset=-0.5  TranslationLengthUnit=m  TranslationStandardAxis=+Y  TranslationCartesianOffset=0  TranslationROffset=0  TranslationROffsetUnits=m  TranslationZOffset=0  TranslationZOffsetUnits=m  TranslationThetaOffset=0  TranslationThetaOffsetUnits=deg  RotationMethod=StandardAxis  RotationAngleUnits=deg  RotationStandardAxis=+X  RotationAngle=90  RotationArbitraryAxis=[0 0 1]  FollAlignAxisA=+X  BaseAlignAxisA=+Y  FollAlignAxisB=+Y  BaseAlignAxisB=+Z  RotationSequenceAxes=BaseAxes  RotationSequence=ZXZ  RotationSequenceAngles=[180 0 0]  RotationSequenceAnglesUnits=deg  RotationMatrix=[1 0 0; 0 1 0; 0 0 1]
  LK Axis Rotation2 : sm_lib/Frames and Transforms/Rigid Transform  TranslationMethod=None  TranslationStandardOffset=-0.5  TranslationLengthUnit=m  TranslationStandardAxis=+Y  TranslationCartesianOffset=0  TranslationROffset=0  TranslationROffsetUnits=m  TranslationZOffset=0  TranslationZOffsetUnits=m  TranslationThetaOffset=0  TranslationThetaOffsetUnits=deg  RotationMethod=StandardAxis  RotationAngleUnits=deg  RotationStandardAxis=+X  RotationAngle=-90  RotationArbitraryAxis=[0 0 1]  FollAlignAxisA=+X  BaseAlignAxisA=+Y  FollAlignAxisB=+Y  BaseAlignAxisB=+Z  RotationSequenceAxes=BaseAxes  RotationSequence=ZXZ  RotationSequenceAngles=[180 0 0]  RotationSequenceAnglesUnits=deg  RotationMatrix=[1 0 0; 0 1 0; 0 0 1]
  Left Hip (LH) Pitch (about X) and Roll (about Y) Joints : sm_lib/Joints/Universal Joint  JointMode=Normal  SenseConstraintForce=off  SenseConstraintForceX=off  SenseConstraintForceY=off  SenseConstraintForceZ=off  SenseConstraintTorque=off  SenseConstraintTorqueX=off  SenseConstraintTorqueY=off  SenseConstraintTorqueZ=off  SenseTotalForce=off  SenseTotalForceX=off  SenseTotalForceY=off  SenseTotalForceZ=off  SenseTotalTorque=off  SenseTotalTorqueX=off  SenseTotalTorqueY=off  SenseTotalTorqueZ=off  CompositeWrenchDir=FollowerOnBase  CompositeWrenchFrame=FollowerFrame  RxEquilibriumPosition=0  RxEquilibriumPositionUnits=deg  RxSpringStiffness=0  RxSpringStiffnessUnits=N*m/deg  RxDampingCoefficient=0  RxDampingCoefficientUnits=N*m/(deg/s)  RxTorqueActuationMode=InputTorque  RxMotionActuationMode=ComputedMotion  RxSensePosition=on  RxSenseVelocity=on  RxSenseAcceleration=on  RxSenseTorqueForce=off  RxSenseLowerLimitTorqueForce=off  RxSenseUpperLimitTorqueForce=off  RxLowerLimitSpecify=off  RxLowerLimitBound=-90  RxLowerLimitBoundUnits=deg  RxLowerLimitStiffness=1e4  RxLowerLimitStiffnessUnits=N*m/deg  RxLowerLimitDamping=10  RxLowerLimitDampingUnits=N*m/(deg/s)  RxLowerLimitTransitionRegionWidth=0.1  RxLowerLimitTransitionRegionWidthUnits=deg  RxUpperLimitSpecify=off  RxUpperLimitBound=90  RxUpperLimitBoundUnits=deg  RxUpperLimitStiffness=1e4  RxUpperLimitStiffnessUnits=N*m/deg  RxUpperLimitDamping=10  RxUpperLimitDampingUnits=N*m/(deg/s)  RxUpperLimitTransitionRegionWidth=0.1  RxUpperLimitTransitionRegionWidthUnits=deg  RxPositionTargetSpecify=on  RxPositionTargetPriority=High  RxPositionTargetValue=ICs.lLeg.hip.qP0  RxPositionTargetValueUnits=rad  RxVelocityTargetSpecify=on  RxVelocityTargetPriority=High  RxVelocityTargetValue=0  RxVelocityTargetValueUnits=rad/s  RyEquilibriumPosition=0  RyEquilibriumPositionUnits=deg  RySpringStiffness=0  RySpringStiffnessUnits=N*m/deg  RyDampingCoefficient=0  RyDampingCoefficientUnits=N*m/(deg/s)  RyTorqueActuationMode=InputTorque  RyMotionActuationMode=ComputedMotion  RySensePosition=on  RySenseVelocity=on  RySenseAcceleration=on  RySenseTorqueForce=off  RySenseLowerLimitTorqueForce=off  RySenseUpperLimitTorqueForce=off  RyLowerLimitSpecify=off  RyLowerLimitBound=-90  RyLowerLimitBoundUnits=deg  RyLowerLimitStiffness=1e4  RyLowerLimitStiffnessUnits=N*m/deg  RyLowerLimitDamping=10  RyLowerLimitDampingUnits=N*m/(deg/s)  RyLowerLimitTransitionRegionWidth=0.1  RyLowerLimitTransitionRegionWidthUnits=deg  RyUpperLimitSpecify=off  RyUpperLimitBound=90  RyUpperLimitBoundUnits=deg  RyUpperLimitStiffness=1e4  RyUpperLimitStiffnessUnits=N*m/deg  RyUpperLimitDamping=10  RyUpperLimitDampingUnits=N*m/(deg/s)  RyUpperLimitTransitionRegionWidth=0.1  RyUpperLimitTransitionRegionWidthUnits=deg  RyPositionTargetSpecify=on  RyPositionTargetPriority=High  RyPositionTargetValue=ICs.lLeg.hip.qR0  RyPositionTargetValueUnits=rad  RyVelocityTargetSpecify=on  RyVelocityTargetPriority=High  RyVelocityTargetValue=0  RyVelocityTargetValueUnits=rad/s
  Left Knee (LK) Pitch : sm_lib/Joints/Revolute Joint  JointMode=Normal  SenseConstraintForce=off  SenseConstraintForceX=off  SenseConstraintForceY=off  SenseConstraintForceZ=off  SenseConstraintTorque=off  SenseConstraintTorqueX=off  SenseConstraintTorqueY=off  SenseConstraintTorqueZ=off  SenseTotalForce=off  SenseTotalForceX=off  SenseTotalForceY=off  SenseTotalForceZ=off  SenseTotalTorque=off  SenseTotalTorqueX=off  SenseTotalTorqueY=off  SenseTotalTorqueZ=off  CompositeWrenchDir=FollowerOnBase  CompositeWrenchFrame=FollowerFrame  EquilibriumPosition=0  EquilibriumPositionUnits=deg  SpringStiffness=0  SpringStiffnessUnits=N*m/deg  DampingCoefficient=0  DampingCoefficientUnits=N*m/(deg/s)  TorqueActuationMode=InputTorque  MotionActuationMode=ComputedMotion  SensePosition=on  SenseVelocity=on  SenseAcceleration=on  SenseTorqueForce=off  SenseLowerLimitTorqueForce=off  SenseUpperLimitTorqueForce=off  LowerLimitSpecify=off  LowerLimitBound=-90  LowerLimitBoundUnits=deg  LowerLimitStiffness=1e4  LowerLimitStiffnessUnits=N*m/deg  LowerLimitDamping=10  LowerLimitDampingUnits=N*m/(deg/s)  LowerLimitTransitionRegionWidth=0.1  LowerLimitTransitionRegionWidthUnits=deg  UpperLimitSpecify=off  UpperLimitBound=90  UpperLimitBoundUnits=deg  UpperLimitStiffness=1e4  UpperLimitStiffnessUnits=N*m/deg  UpperLimitDamping=10  UpperLimitDampingUnits=N*m/(deg/s)  UpperLimitTransitionRegionWidth=0.1  UpperLimitTransitionRegionWidthUnits=deg  PositionTargetSpecify=on  PositionTargetPriority=High  PositionTargetValue=ICs.lLeg.knee.qP0  PositionTargetValueUnits=rad  VelocityTargetSpecify=on  VelocityTargetPriority=High  VelocityTargetValue=0  VelocityTargetValueUnits=rad/s
  Mux1 : Mux  Inputs=5
  Mux2 : Mux  Inputs=5
  Mux7 : Mux  Inputs=5
  Rotation Sensor Knee : Subsystem
  Selector1 : Selector  InputPortWidth=3  IndexOptions=Index vector (dialog)  Indices=[2]  OutputSizes=1
  Sensor Left Ankle : Subsystem
  Shank : Subsystem
  Stop Simulation1 : Stop
  Sum{1..2,4..5} (4 alike) : Sum  Inputs=|++
  Terminator : Terminator
  Thigh : Subsystem
  Universal Joint : sm_lib/Joints/Universal Joint  JointMode=Normal  SenseConstraintForce=off  SenseConstraintForceX=off  SenseConstraintForceY=off  SenseConstraintForceZ=off  SenseConstraintTorque=off  SenseConstraintTorqueX=off  SenseConstraintTorqueY=off  SenseConstraintTorqueZ=off  SenseTotalForce=off  SenseTotalForceX=off  SenseTotalForceY=off  SenseTotalForceZ=off  SenseTotalTorque=off  SenseTotalTorqueX=off  SenseTotalTorqueY=off  SenseTotalTorqueZ=off  CompositeWrenchDir=FollowerOnBase  CompositeWrenchFrame=BaseFrame  RxEquilibriumPosition=0  RxEquilibriumPositionUnits=deg  RxSpringStiffness=0  RxSpringStiffnessUnits=N*m/deg  RxDampingCoefficient=0  RxDampingCoefficientUnits=N*m/(deg/s)  RxTorqueActuationMode=InputTorque  RxMotionActuationMode=ComputedMotion  RxSensePosition=on  RxSenseVelocity=on  RxSenseAcceleration=on  RxSenseTorqueForce=off  RxSenseLowerLimitTorqueForce=off  RxSenseUpperLimitTorqueForce=off  RxLowerLimitSpecify=off  RxLowerLimitBound=-90  RxLowerLimitBoundUnits=deg  RxLowerLimitStiffness=1e4  RxLowerLimitStiffnessUnits=N*m/deg  RxLowerLimitDamping=10  RxLowerLimitDampingUnits=N*m/(deg/s)  RxLowerLimitTransitionRegionWidth=0.1  RxLowerLimitTransitionRegionWidthUnits=deg  RxUpperLimitSpecify=off  RxUpperLimitBound=90  RxUpperLimitBoundUnits=deg  RxUpperLimitStiffness=1e4  RxUpperLimitStiffnessUnits=N*m/deg  RxUpperLimitDamping=10  RxUpperLimitDampingUnits=N*m/(deg/s)  RxUpperLimitTransitionRegionWidth=0.1  RxUpperLimitTransitionRegionWidthUnits=deg  RxPositionTargetSpecify=on  RxPositionTargetPriority=High  RxPositionTargetValue=0  RxPositionTargetValueUnits=rad  RxVelocityTargetSpecify=on  RxVelocityTargetPriority=High  RxVelocityTargetValue=0  RxVelocityTargetValueUnits=deg/s  RyEquilibriumPosition=0  RyEquilibriumPositionUnits=deg  RySpringStiffness=0  RySpringStiffnessUnits=N*m/deg  RyDampingCoefficient=0  RyDampingCoefficientUnits=N*m/(deg/s)  RyTorqueActuationMode=InputTorque  RyMotionActuationMode=ComputedMotion  RySensePosition=on  RySenseVelocity=on  RySenseAcceleration=on  RySenseTorqueForce=off  RySenseLowerLimitTorqueForce=off  RySenseUpperLimitTorqueForce=off  RyLowerLimitSpecify=off  RyLowerLimitBound=-90  RyLowerLimitBoundUnits=deg  RyLowerLimitStiffness=1e4  RyLowerLimitStiffnessUnits=N*m/deg  RyLowerLimitDamping=10  RyLowerLimitDampingUnits=N*m/(deg/s)  RyLowerLimitTransitionRegionWidth=0.1  RyLowerLimitTransitionRegionWidthUnits=deg  RyUpperLimitSpecify=off  RyUpperLimitBound=90  RyUpperLimitBoundUnits=deg  RyUpperLimitStiffness=1e4  RyUpperLimitStiffnessUnits=N*m/deg  RyUpperLimitDamping=10  RyUpperLimitDampingUnits=N*m/(deg/s)  RyUpperLimitTransitionRegionWidth=0.1  RyUpperLimitTransitionRegionWidthUnits=deg  RyPositionTargetSpecify=on  RyPositionTargetPriority=High  RyPositionTargetValue=-ICs.lLeg.ankle.qP0  RyPositionTargetValueUnits=rad  RyVelocityTargetSpecify=off  RyVelocityTargetPriority=High  RyVelocityTargetValue=0  RyVelocityTargetValueUnits=deg/s
  extension definition : Gain  Gain=-1
  extension definition1 : Gain  Gain=-1
  extension definition2 : Gain  Gain=-1
  extensor definition : Gain  Gain=-1
  Left Hip : PMIOPort  Side=Left
  Left Heel : PMIOPort  Port=2  Side=Right
  Left Ball : PMIOPort  Port=3  Side=Right
  Right Ball : PMIOPort  Port=4  Side=Right
  Right Heel : PMIOPort  Port=5  Side=Right
  Rotation Matrix Left Knee (world) : Outport
  " Position Left Ankle [m]" : Outport  Port=2
  Joint Angles Left [rad] : Outport  Port=3
  "Joint Velocities Left [rad/s] " : Outport  Port=4
  Joint Accelerations Left [rad/s^2] : Outport  Port=5
  tag scope: AnklePosL=global
  wires:
  extension definition1/1 -> Mux1/5, Ankle Mechanical Limits/1(dq [rad/s])
  AP Pos Sensor/1 -> extension definition/1
  Ankle Mechanical Limits/1(tau [Nm]) -> Sum2/2
  AP Vel Sensor/1 -> extension definition1/1
  Sum2/1 -> extensor definition/1
  "H Roll Vel Sensor "/1 -> Mux1/2, Hip Roll Mechanical Limits/1(dq [rad/s])
  K Vel Sensor/1 -> Mux1/3, Knee Mechanical Limits/1(dq [rad/s])
  Knee Mechanical Limits/1(tau [Nm]) -> Sum5/2
  Hip Roll Mechanical Limits/1(tau [Nm]) -> Sum1/2
  H Pitch Vel Sensor/1 -> Mux1/1, Hip Pitch Mechanical Limits/1(dq [rad/s])
  Hip Pitch Mechanical Limits/1(tau [Nm]) -> Sum4/2
  Sum4/1 -> H Pitch Actuator/1
  Sum1/1 -> H Roll Actuator/1
  Sum5/1 -> " K Actuator"/1
  extensor definition/1 -> A Actuator/1
  Mux1/1 -> "Joint Velocities Left [rad/s] "/1
  Mux2/1 -> Joint Accelerations Left [rad/s^2]/1
  H Pitch Acc Sensor/1 -> Mux2/1
  H Roll Acc Sensor/1 -> Mux2/2
  K Acc Sensor/1 -> Mux2/3
  AP acc Sensor/1 -> extension definition2/1
  extension definition2/1 -> Mux2/5
  Demux/1 -> Sum4/1
  Demux/2 -> Sum1/1
  Demux/3 -> Sum5/1
  Demux/4 -> A Actuator1/1
  Sensor Left Ankle/1(Position [m]) -> " Position Left Ankle [m]"/1, Selector1/1, [AnklePosL]
  Rotation Sensor Knee/1(Rotation Matrix) -> Rotation Matrix Left Knee (world)/1
  Sensor Left Ankle/2(Velocity [m/s]) -> Terminator/1
  Torques [Nm]/1 -> Demux/1
  K Pos Sensor/1 -> Mux7/3, Knee Mechanical Limits/2(q [rad])  "qK"
  H Pitch Pos Sensor/1 -> Hip Pitch Mechanical Limits/2(q [rad]), Mux7/1  "qHP"
  H Roll Pos Sensor/1 -> Mux7/2, Hip Roll Mechanical Limits/2(q [rad])  "qHR"
  extension definition/1 -> Ankle Mechanical Limits/2(q [rad]), Mux7/5  "qA"
  Mux7/1 -> Joint Angles Left [rad]/1
  Selector1/1 -> Compare To Constant1/1
  Compare To Constant1/1 -> Stop Simulation1/1
  AR Vel Sensor/1 -> Mux1/4
  AR acc Sensor/1 -> Mux2/4
  AR Pos Sensor/1 -> Mux7/4
  Demux/5 -> Sum2/1
  Constant/1 -> A Actuator2/1
  connections:
  LK Axis Rotation2/RConn1 -- Sensor Left Ankle/LConn1 -- Foot/LConn1
  Left Hip (LH) Pitch (about X) and Roll (about Y) Joints/RConn1 -- LH Axis Inverse Rotation/LConn1
  Thigh/RConn1 -- Rotation Sensor Knee/LConn1 -- LK Axis Rotation/LConn1
  Shank/LConn1 -- Left Knee (LK) Pitch/RConn1
  Left Hip (LH) Pitch (about X) and Roll (about Y) Joints/LConn1 -- LH Axis Rotation/RConn1
  H Pitch Vel Sensor/LConn1 -- Left Hip (LH) Pitch (about X) and Roll (about Y) Joints/RConn3
  H Pitch Pos Sensor/LConn1 -- Left Hip (LH) Pitch (about X) and Roll (about Y) Joints/RConn2
  K Pos Sensor/LConn1 -- Left Knee (LK) Pitch/RConn2
  K Vel Sensor/LConn1 -- Left Knee (LK) Pitch/RConn3
  LH Axis Rotation/LConn1 -- Left Hip/RConn1
  Left Hip (LH) Pitch (about X) and Roll (about Y) Joints/RConn6 -- "H Roll Vel Sensor "/LConn1
  Left Hip (LH) Pitch (about X) and Roll (about Y) Joints/RConn5 -- H Roll Pos Sensor/LConn1
  Left Hip (LH) Pitch (about X) and Roll (about Y) Joints/RConn4 -- H Pitch Acc Sensor/LConn1
  Left Hip (LH) Pitch (about X) and Roll (about Y) Joints/RConn7 -- H Roll Acc Sensor/LConn1
  Left Knee (LK) Pitch/RConn4 -- K Acc Sensor/LConn1
  LK Axis Rotation/RConn1 -- Left Knee (LK) Pitch/LConn1
  Right Heel/RConn1 -- Foot/LConn3
  Foot/LConn2 -- Left Heel/RConn1
  Left Ball/RConn1 -- Foot/RConn1
  Right Ball/RConn1 -- Foot/RConn2
  Thigh/LConn1 -- LH Axis Inverse Rotation/RConn1
  " K Actuator"/RConn1 -- Left Knee (LK) Pitch/LConn2
  H Pitch Actuator/RConn1 -- Left Hip (LH) Pitch (about X) and Roll (about Y) Joints/LConn2
  H Roll Actuator/RConn1 -- Left Hip (LH) Pitch (about X) and Roll (about Y) Joints/LConn3
  Universal Joint/LConn1 -- LK Axis Rotation1/RConn1
  Universal Joint/RConn1 -- LK Axis Rotation2/LConn1
  Universal Joint/RConn5 -- AP Pos Sensor/LConn1
  Universal Joint/RConn6 -- AP Vel Sensor/LConn1
  Universal Joint/RConn7 -- AP acc Sensor/LConn1
  Shank/RConn1 -- LK Axis Rotation1/LConn1
  Universal Joint/RConn4 -- AR acc Sensor/LConn1
  Universal Joint/RConn3 -- AR Vel Sensor/LConn1
  Universal Joint/RConn2 -- AR Pos Sensor/LConn1
  A Actuator/RConn1 -- Universal Joint/LConn3
  A Actuator1/RConn1 -- Universal Joint/LConn2
